simulink model "motore"  (R2022a)
settings: Solver=ode45  StartTime=0.0  StopTime=0.5  MaxStep=0.001  RelTol=1e-3
values from neighbouring files (symbols this model uses):
  rads2rpm = 60 / (2 * pi)    (= 9.54929658551)    [simulink_motore.m]
  Ts = 0.01    [simulink_motore.m]
undefined symbols (not defined in the file or in its folder): DiscIntNeverNeededParam, drv, mot, wctrl
settings Model: Creator=loren  LastModifiedBy=loren

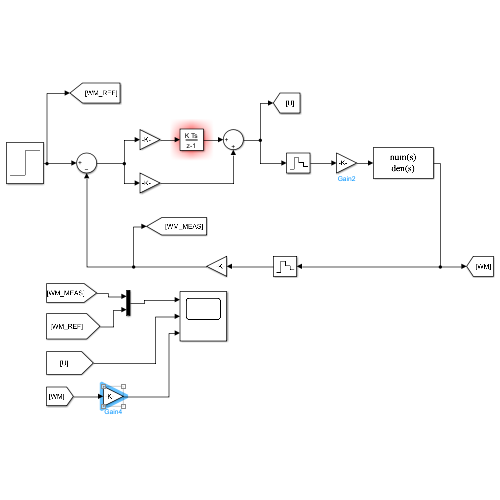
[thumbnail: Simulink's stored preview of the top-level diagram]
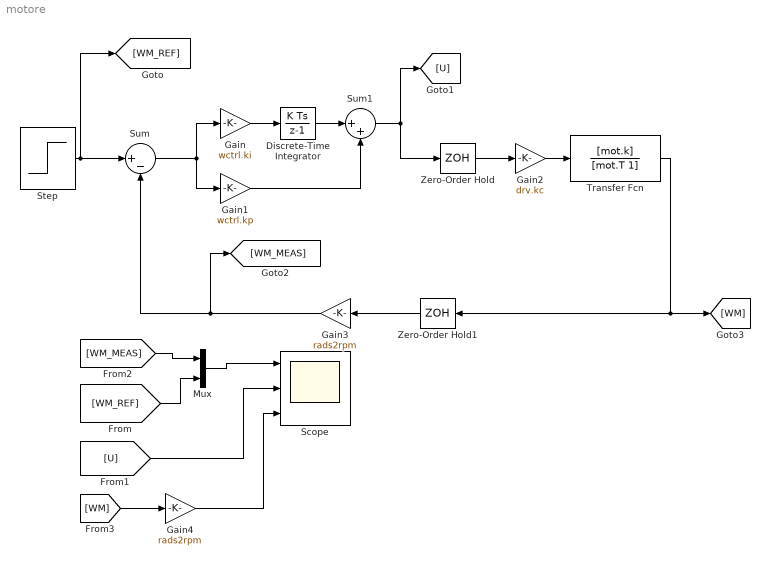
== system motore ==
  Discrete-Time Integrator : DiscreteIntegrator  SampleTime=Ts  ICPrevOutput=DiscIntNeverNeededParam  ICPrevScaledInput=DiscIntNeverNeededParam
  Gain : Gain  Gain=wctrl.ki
  Gain1 : Gain  Gain=wctrl.kp
  Gain2 : Gain  Gain=drv.kc
  Gain3 : Gain  Gain=rads2rpm
  Gain4 : Gain  Gain=rads2rpm
  Mux : Mux  Inputs=2
  Scope : Scope  NumInputPorts=3
  Step : Step  Time=0  After=300  SampleTime=0
  Sum : Sum  Inputs=|+-
  Sum1 : Sum  Inputs=|++
  Transfer Fcn : TransferFcn  Numerator=[mot.k]  Denominator=[mot.T 1]
  Zero-Order Hold : ZeroOrderHold  SampleTime=Ts
  Zero-Order Hold1 : ZeroOrderHold  SampleTime=Ts
  wires:
  Step/1 -> [WM_REF], Sum/1
  Gain/1 -> Discrete-Time Integrator/1
  Sum/1 -> Gain/1, Gain1/1
  Discrete-Time Integrator/1 -> Sum1/1
  Gain1/1 -> Sum1/2
  Sum1/1 -> [U], Zero-Order Hold/1
  Gain2/1 -> Transfer Fcn/1
  Transfer Fcn/1 -> [WM], Zero-Order Hold1/1
  Gain3/1 -> [WM_MEAS], Sum/2
  [WM_MEAS] -> Mux/1
  [WM_REF] -> Mux/2
  Mux/1 -> Scope/1
  [U] -> Scope/2
  Zero-Order Hold/1 -> Gain2/1
  Zero-Order Hold1/1 -> Gain3/1
  [WM] -> Gain4/1
  Gain4/1 -> Scope/3
